simulink model "ejercicio1_1"  (R2022b)
settings: Solver=VariableStepAuto  StartTime=0.0  StopTime=5  RelTol=1e-3
values from neighbouring files (symbols this model uses):
  g = 9.81    [ejercicio.m]
  l1 = 0.3    [ejercicio.m]
  l2 = 0.25    [ejercicio.m]
  m1 = 0.2    [ejercicio.m]
  m2 = 0.1    [ejercicio.m]
settings Model: Creator=mluser  LastModifiedBy=mluser

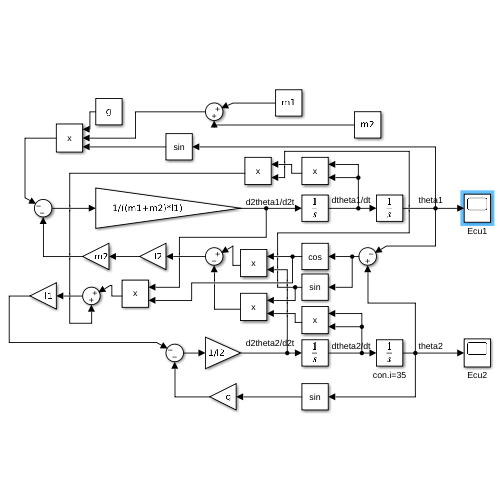
[thumbnail: Simulink's stored preview of the top-level diagram]
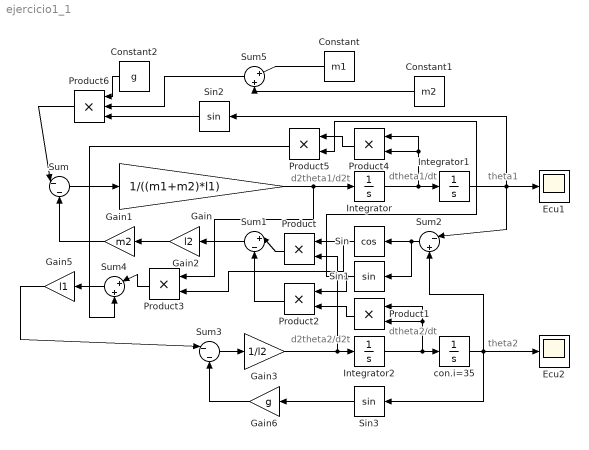
== system ejercicio1_1 ==
  note: theta1
  note: dtheta1/dt
  note: d2theta1/d2t
  note: dtheta2/dt
  note: d2theta2/d2t
  note: theta2
  Constant : Constant  Value=m1
  Constant1 : Constant  Value=m2
  Constant2 : Constant  Value=g
  Ecu1 : Scope
  Ecu2 : Scope
  Gain : Gain  Gain=1/((m1+m2)*l1)
  Gain1 : Gain  Gain=m2
  Gain2 : Gain  Gain=l2
  Gain3 : Gain  Gain=1/l2
  Gain5 : Gain  Gain=l1
  Gain6 : Gain  Gain=g
  Integrator : Integrator
  Integrator1 : Integrator
  Integrator2 : Integrator
  Product{,1..5} (6 alike) : Product
  Product6 : Product  Inputs=3
  Sin : Trigonometry  Operator=cos
  Sin1 : Trigonometry
  Sin2 : Trigonometry
  Sin3 : Trigonometry
  Sum : Sum  Inputs=|-|-
  Sum1 : Sum  Inputs=|+|-
  Sum2 : Sum  Inputs=|-|+
  Sum3 : Sum  Inputs=|-|-
  Sum4 : Sum  Inputs=|+|+
  Sum5 : Sum  Inputs=|+|+
  con.i=35 : Integrator  InitialCondition=(35*pi)/180
  wires:
  Integrator1/1 -> Sin2/1, Sum2/1, Ecu1/1
  Integrator2/1 -> Product1/1, Product1/2, con.i=35/1
  Gain3/1 -> Product/2, Integrator2/1
  con.i=35/1 -> Sin3/1, Ecu2/1, Sum2/2
  Gain/1 -> Product3/1, Integrator/1
  Sum/1 -> Gain/1
  Gain1/1 -> Sum/2
  Gain2/1 -> Gain1/1
  Sum1/1 -> Gain2/1
  Sum2/1 -> Sin1/1, Sin/1
  Sin/1 -> Product3/2, Product/1
  Product/1 -> Sum1/1
  Product1/1 -> Product2/2
  Sin1/1 -> Product2/1, Product5/2
  Product2/1 -> Sum1/2
  Sin2/1 -> Product6/3
  Product6/1 -> Sum/1
  Sum3/1 -> Gain3/1
  Gain5/1 -> Sum3/1
  Product3/1 -> Sum4/1
  Integrator/1 -> Product4/2, Product4/1, Integrator1/1
  Product4/1 -> Product5/1
  Product5/1 -> Sum4/2
  Sum4/1 -> Gain5/1
  Gain6/1 -> Sum3/2
  Sin3/1 -> Gain6/1
  Constant/1 -> Sum5/1
  Constant1/1 -> Sum5/2
  Constant2/1 -> Product6/1
  Sum5/1 -> Product6/2
